simulink model "tank_circuit"  (R2019a)
settings: Solver=VariableStepAuto  StartTime=0.0  StopTime=10e-3  RelTol=1e-3
StopFcn:
  | ee_addSimlogTimeStamp(bdroot)
CloseFcn:
  | try,close(h1_ee_radio_am_receiver),end
  | clear h1_ee_radio_am_receiver
  | 
  | clear simlog_ee_radio_am_receiver
  | clear logsout_ee_radio_am_receiver
Description:
  | AM Radio Receiver
settings Model: Creator=The MathWorks, Inc.  LastModifiedBy=donald.taylor2
settings DataIOCC: MaxDataPoints=135000  SaveOutput=off  SignalLogging=off  DSMLogging=off  SaveTime=off  ReturnWorkspaceOutputs=off  SignalLoggingName=logsout_ee_radio_am_receiver
settings DebuggingCC: PregeneratedLibrarySubsystemCodeDiagnostic=none  ArithmeticOperatorsInVariantConditions=warning
settings SFSimCC: SimUseLocalCustomCode=off
settings RTWCC: RTWUseLocalCustomCode=off
settings CodeAppCC: StateflowObjectComments=on
settings GRTTargetCC: TargetLangStandard=C89/C90 (ANSI)
settings ConfigComp: CovMetricSettings=dsw  CovHtmlReporting=on  CovSaveCumulativeToWorkspaceVar=on  CovSaveSingleToWorkspaceVar=on  CovShowResultsExplorer=off  CovExternalEMLEnable=off
settings SimscapeCC: SimscapeLogType=all  SimscapeLogSimulationStatistics=on  SimscapeLogName=simlog_ee_radio_am_receiver  SimscapeLogDataHistory=135000

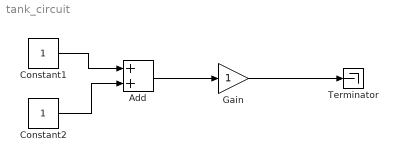
== system tank_circuit ==
  Add : Sum
  Constant1 : Constant
  Constant2 : Constant
  Gain : Gain
  Terminator : Terminator
  wires:
  Constant1/1 -> Add/1
  Constant2/1 -> Add/2
  Add/1 -> Gain/1
  Gain/1 -> Terminator/1
